simulink model "buckwthsaw"  (R2014a)
settings: Solver=ode23tb  StartTime=0.0  StopTime=0.05  RelTol=1e-3
libraries: powerlib x11, simulink x1
settings Model: Creator=Zaid  LastModifiedBy=Zaid

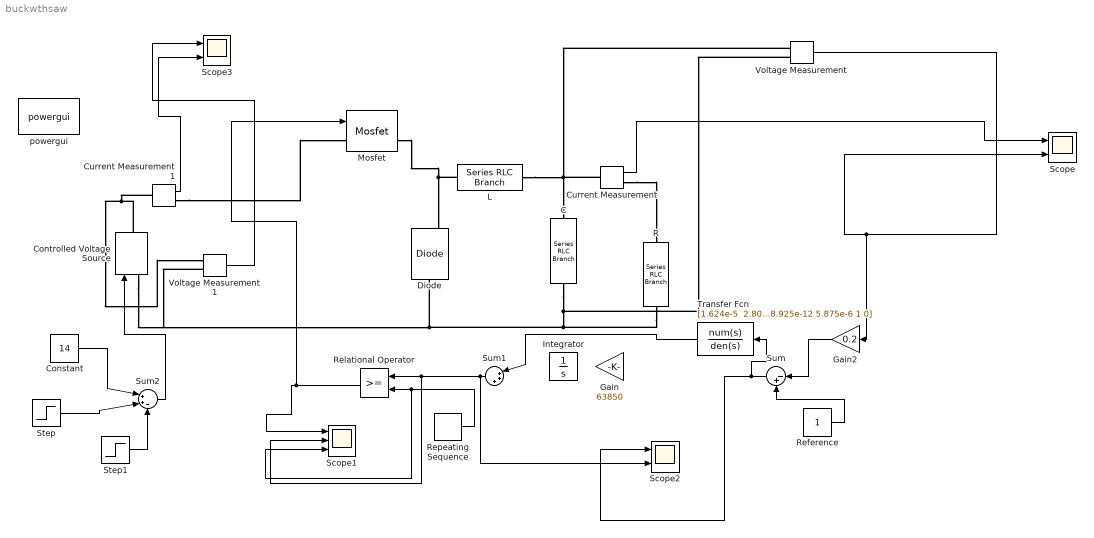
== system buckwthsaw ==
  C : powerlib/Elements/Series RLC Branch  LConnTagsString=__new0  RConnTagsString=__new0  BranchType=RC  Resistance=0.1  Inductance=327e-6  SetiL0=off  InitialCurrent=0  Capacitance=750e-9  Setx0=off  InitialVoltage=0  Measurements=None
  Constant : Constant  Value=14
  Controlled Voltage Source : powerlib/Electrical Sources/Controlled Voltage Source  Initialize=on  Source_Type=AC  Amplitude=0  Phase=0  Frequency=0  Measurements=None
  Current Measurement : powerlib/Measurements/Current Measurement  PhasorSimulation=off  OutputType=Complex  PSBequivalent=0
  Current Measurement1 : powerlib/Measurements/Current Measurement  PhasorSimulation=off  OutputType=Complex  PSBequivalent=0
  Diode : powerlib/Power Electronics/Diode  Ron=0.001  Lon=0  Vf=0.55  IC=0  UseSnubber=off  Rs=500  Cs=250e-9  Measurements=on
  Gain : Gain  Gain=63850
  Gain2 : Gain  Gain=0.2
  Integrator : Integrator
  L : powerlib/Elements/Series RLC Branch  LConnTagsString=__new0  RConnTagsString=__new0  BranchType=RL  Resistance=0.001  Inductance=109.195e-6  SetiL0=off  InitialCurrent=0  Capacitance=1e-6  Setx0=off  InitialVoltage=0  Measurements=None
  Mosfet : powerlib/Power Electronics/Mosfet  Ron=0.15  Lon=12  Rd=0.01  Vfd=1.3  IC=0  Rs=1e5  Cs=inf  Measurements=on
  R : powerlib/Elements/Series RLC Branch  LConnTagsString=__new0  RConnTagsString=__new0  BranchType=R  Resistance=5  Inductance=327e-6  SetiL0=off  InitialCurrent=0  Capacitance=1.25e-8  Setx0=off  InitialVoltage=0  Measurements=None
  Reference : Constant
  Relational Operator : RelationalOperator  OutDataTypeStr=boolean  ZeroCross=off
  Repeating Sequence : simulink/Sources/Repeating Sequence  rep_seq_t=[0 1/100000]  rep_seq_y=[0 3]
  Scope : Scope  NumInputPorts=2
      settings: YMin=0.99955~4.99775  YMax=1.0004~5.002
  Scope1 : Scope  NumInputPorts=3
      settings: YMin=0~18.995~0  YMax=1~19.0325~50
  Scope2 : Scope  NumInputPorts=2
      settings: TimeRange=5.802849055690316e-05  YMin=-0.5~0.9832304526748972  YMax=2.5~1.211488340192044  SaveName=ScopeData2
  Scope3 : Scope  NumInputPorts=2
      settings: YMin=0.85~4.2  YMax=1.15~5.7  SaveName=ScopeData3
  Step : Step  Time=0.02  After=0.5  SampleTime=0
  Step1 : Step  Time=0.04  After=1.9  SampleTime=0
  Sum : Sum  Inputs=|-+
  Sum1 : Sum  Inputs=|+++
  Sum2 : Sum  Inputs=|++-
  Transfer Fcn : TransferFcn  Numerator="[1.624e-5  2.805  1.211e5]"  Denominator=[8.925e-12 5.875e-6 1 0]
  Voltage Measurement : powerlib/Measurements/Voltage Measurement  PhasorSimulation=off  OutputType=Complex  PSBequivalent=0
  Voltage Measurement1 : powerlib/Measurements/Voltage Measurement  PhasorSimulation=off  OutputType=Complex  PSBequivalent=0
  powergui : powerlib/powergui  Priority=1  SimulationMode=Discrete  SolverType=Tustin  SampleTime=1e-8  frequency=60  SPID=off  DisableSnubberDevices=off  DisableRonSwitches=off  DisableVfSwitches=off  SwTol=0  Interpol=off  DisplayEquations=off  Ts=0  methode=off  frequencyindice=0  Pbase=100e6  ErrMax=1e-4  Iterations=50  UnitsV=kV  UnitsW=MW  FunctionMessages=off  echomessages=off  HookPort=off  EnableUseOfTLC=off  x0status=blocks  RestoreLinks=warning  ResistiveCurrentMeasurement=off  Frange=[0:2:500]  Ylog=off  Xlog=on  ShowGrid=off  save=off  variable=ZData  structure=0  ZoomFFT=off  StartTime=0.0  cycles=1  DisplayStyle=1  fundamental=60  FreqAxis=off  MaxFrequency=1000  frequencyindicesteady=1  RmsSteady=1  display=off
  wires:
  Voltage Measurement/1 -> Gain2/1, Scope/2
  Reference/1 -> Sum/2
  Sum/1 -> Transfer Fcn/1, Scope2/1
  Repeating Sequence/1 -> Scope1/3, Relational Operator/2
  Relational Operator/1 -> Mosfet/1, Scope1/1
  Sum1/1 -> Scope1/2, Relational Operator/1, Scope2/2
  Constant/1 -> Sum2/1
  Sum2/1 -> Controlled Voltage Source/1
  Voltage Measurement1/1 -> Scope3/1
  Current Measurement1/1 -> Scope3/2
  Transfer Fcn/1 -> Sum1/1
  Current Measurement/1 -> Scope/1
  Step/1 -> Sum2/2
  Step1/1 -> Sum2/3
  Gain2/1 -> Sum/1
  connections:
  Controlled Voltage Source/RConn1 -- Current Measurement1/LConn1 -- Voltage Measurement1/LConn1
  L/LConn1 -- Mosfet/RConn1 -- Diode/RConn1
  C/RConn1 -- Voltage Measurement/LConn2 -- R/RConn1 -- Voltage Measurement1/LConn2 -- Controlled Voltage Source/LConn1 -- Diode/LConn1
  Current Measurement1/RConn1 -- Mosfet/LConn1
  L/RConn1 -- Current Measurement/LConn1 -- Voltage Measurement/LConn1 -- C/LConn1
  Current Measurement/RConn1 -- R/LConn1
